simulink model "Simulation2"  (R2023b)
settings: Solver=VariableStepAuto  StartTime=0.0  StopTime=5  RelTol=1e-3
values from neighbouring files (symbols this model uses):
  Adj = Adj1'    [graph_plot.m]
  G = digraph(Adj)    [graph_plot.m]
undefined symbols (not defined in the file or in its folder): A, B, c, C, F, K, Ko, L1, x0_0, xi_0
libraries: simulink x7
settings Model: Creator=fedpa  LastModifiedBy=fedpa

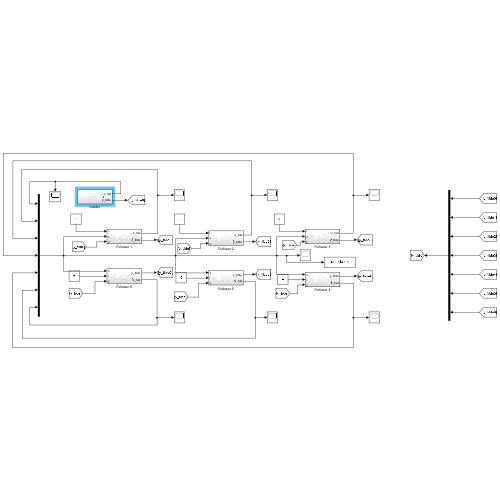
[thumbnail: Simulink's stored preview of the top-level diagram]
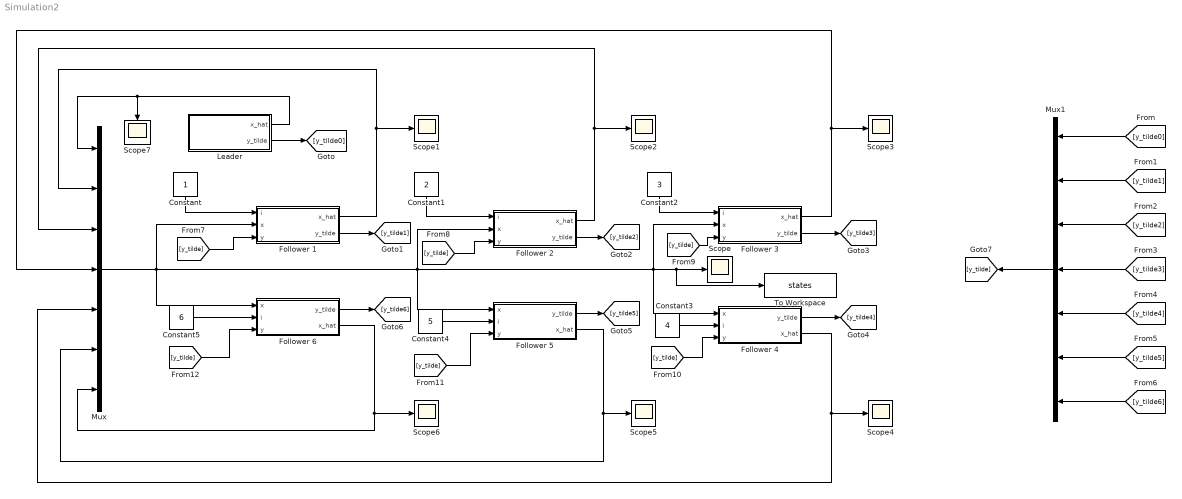
== system Simulation2 ==
  Constant : Constant
  Constant1 : Constant  Value=2
  Constant2 : Constant  Value=3
  Constant3 : Constant  Value=4
  Constant4 : Constant  Value=5
  Constant5 : Constant  Value=6
  Follower 1 : Subsystem
  Follower 2 : Subsystem
  Follower 3 : Subsystem
  Follower 4 : Subsystem
  Follower 5 : Subsystem
  Follower 6 : Subsystem
  Leader : Subsystem
  Mux : Mux  Inputs=7
  Mux1 : Mux  Inputs=7
  Scope{,1..7} (8 alike) : Scope
  To Workspace : ToWorkspace  VariableName=states  SaveFormat=Timeseries  SampleTime=-1
  wires:
  Follower 1/1(x_hat) -> Scope1/1, Mux/2
  Follower 2/1(x_hat) -> Scope2/1, Mux/3
  Follower 3/1(x_hat) -> Scope3/1, Mux/4
  Follower 6/2(x_hat) -> Scope6/1, Mux/7
  Follower 4/2(x_hat) -> Scope4/1, Mux/5
  Mux/1 -> To Workspace/1, Scope/1, Follower 4/1(x), Follower 3/2(x), Follower 5/1(x), Follower 2/2(x), Follower 6/1(x), Follower 1/2(x)
  Constant/1 -> Follower 1/1(i)
  Constant1/1 -> Follower 2/1(i)
  Constant2/1 -> Follower 3/1(i)
  Leader/1(x_hat) -> Scope7/1, Mux/1
  Leader/2(y_tilde) -> [y_tilde0]
  [y_tilde0] -> Mux1/1
  [y_tilde1] -> Mux1/2
  Follower 1/2(y_tilde) -> [y_tilde1]
  Follower 2/2(y_tilde) -> [y_tilde2]
  Follower 3/2(y_tilde) -> [y_tilde3]
  [y_tilde2] -> Mux1/3
  [y_tilde5] -> Mux1/6
  [y_tilde4] -> Mux1/5
  [y_tilde3] -> Mux1/4
  Follower 4/1(y_tilde) -> [y_tilde4]
  Follower 5/2(x_hat) -> Mux/6, Scope5/1
  Follower 5/1(y_tilde) -> [y_tilde5]
  Follower 6/1(y_tilde) -> [y_tilde6]
  [y_tilde6] -> Mux1/7
  Mux1/1 -> [y_tilde]
  [y_tilde] -> Follower 6/3(y)
  [y_tilde] -> Follower 5/3(y)
  [y_tilde] -> Follower 4/3(y)
  [y_tilde] -> Follower 3/3(y)
  [y_tilde] -> Follower 2/3(y)
  [y_tilde] -> Follower 1/3(y)
  Constant4/1 -> Follower 5/2(i)
  Constant5/1 -> Follower 6/2(i)
  Constant3/1 -> Follower 4/2(i)

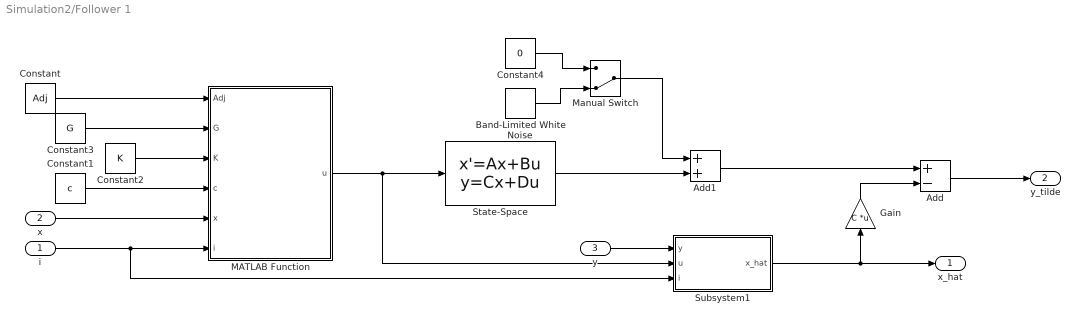
== system Simulation2/Follower 1 ==
  i : Inport
  x : Inport  Port=2
  y : Inport  Port=3
  Add : Sum  Inputs=+-
  Add1 : Sum
  Band-Limited White Noise : simulink/Sources/Band-Limited White Noise  Cov=dis  Ts=0.1  seed=[23341]
  Constant : Constant  Value=Adj  VectorParams1D=off
  Constant1 : Constant  Value=c
  Constant2 : Constant  Value=K  VectorParams1D=off
  Constant3 : Constant  Value=G
  Constant4 : Constant  Value=0
  Gain : Gain  Gain=C  Multiplication=Matrix(K*u)
  MATLAB Function : MATLAB Function  TreatAsAtomicUnit=on
  Manual Switch : ManualSwitch  CurrentSetting=0
  State-Space : StateSpace  A=A-B*Ko  B=B  C=C  D=0  InitialCondition=xi_0
  Subsystem1 : Subsystem
  x_hat : Outport
  y_tilde : Outport  Port=2
  wires:
  x/1 -> MATLAB Function/5(x)
  i/1 -> Subsystem1/3(i), MATLAB Function/6(i)
  Constant/1 -> MATLAB Function/1(Adj)
  Constant1/1 -> MATLAB Function/4(c)
  Constant2/1 -> MATLAB Function/3(K)
  Constant3/1 -> MATLAB Function/2(G)
  MATLAB Function/1(u) -> Subsystem1/2(u), State-Space/1
  Subsystem1/1(x_hat) -> x_hat/1, Gain/1
  Add/1 -> y_tilde/1
  y/1 -> Subsystem1/1(y)
  Gain/1 -> Add/2
  Add1/1 -> Add/1
  Constant4/1 -> Manual Switch/1
  Band-Limited White Noise/1 -> Manual Switch/2
  State-Space/1 -> Add1/2
  Manual Switch/1 -> Add1/1

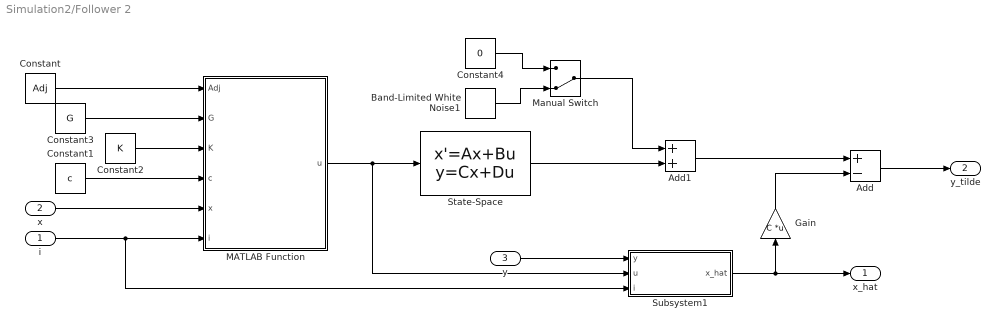
== system Simulation2/Follower 2 ==
  i : Inport
  x : Inport  Port=2
  y : Inport  Port=3
  Add : Sum  Inputs=+-
  Add1 : Sum
  Band-Limited White Noise1 : simulink/Sources/Band-Limited White Noise  Cov=dis  Ts=0.1  seed=[23341]
  Constant : Constant  Value=Adj  VectorParams1D=off
  Constant1 : Constant  Value=c
  Constant2 : Constant  Value=K  VectorParams1D=off
  Constant3 : Constant  Value=G
  Constant4 : Constant  Value=0
  Gain : Gain  Gain=C  Multiplication=Matrix(K*u)
  MATLAB Function : MATLAB Function  TreatAsAtomicUnit=on
  Manual Switch : ManualSwitch  CurrentSetting=0
  State-Space : StateSpace  A=A-B*Ko  B=B  C=C  D=0  InitialCondition=xi_0
  Subsystem1 : Subsystem
  x_hat : Outport
  y_tilde : Outport  Port=2
  wires:
  x/1 -> MATLAB Function/5(x)
  i/1 -> Subsystem1/3(i), MATLAB Function/6(i)
  Constant/1 -> MATLAB Function/1(Adj)
  Constant1/1 -> MATLAB Function/4(c)
  Constant2/1 -> MATLAB Function/3(K)
  Constant3/1 -> MATLAB Function/2(G)
  MATLAB Function/1(u) -> State-Space/1, Subsystem1/2(u)
  Subsystem1/1(x_hat) -> Gain/1, x_hat/1
  Add/1 -> y_tilde/1
  y/1 -> Subsystem1/1(y)
  Gain/1 -> Add/2
  Add1/1 -> Add/1
  Constant4/1 -> Manual Switch/1
  Band-Limited White Noise1/1 -> Manual Switch/2
  State-Space/1 -> Add1/2
  Manual Switch/1 -> Add1/1

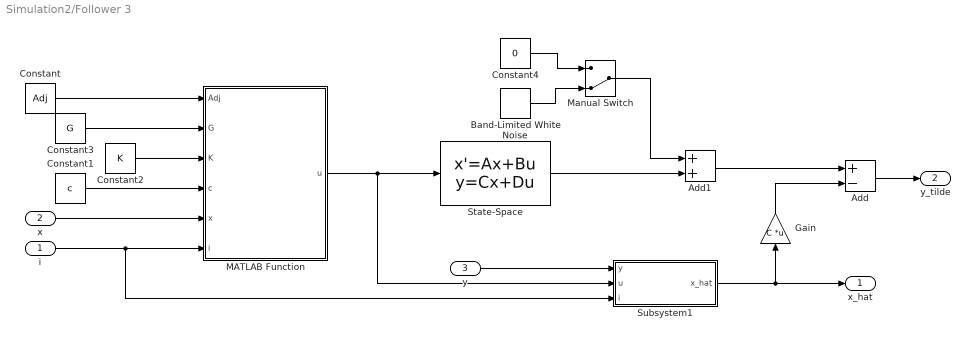
== system Simulation2/Follower 3 ==
  i : Inport
  x : Inport  Port=2
  y : Inport  Port=3
  Add : Sum  Inputs=+-
  Add1 : Sum
  Band-Limited White Noise : simulink/Sources/Band-Limited White Noise  Cov=dis  Ts=0.1  seed=[23341]
  Constant : Constant  Value=Adj  VectorParams1D=off
  Constant1 : Constant  Value=c
  Constant2 : Constant  Value=K  VectorParams1D=off
  Constant3 : Constant  Value=G
  Constant4 : Constant  Value=0
  Gain : Gain  Gain=C  Multiplication=Matrix(K*u)
  MATLAB Function : MATLAB Function  TreatAsAtomicUnit=on
  Manual Switch : ManualSwitch  CurrentSetting=0
  State-Space : StateSpace  A=A-B*Ko  B=B  C=C  D=0  InitialCondition=xi_0
  Subsystem1 : Subsystem
  x_hat : Outport
  y_tilde : Outport  Port=2
  wires:
  x/1 -> MATLAB Function/5(x)
  i/1 -> Subsystem1/3(i), MATLAB Function/6(i)
  Constant/1 -> MATLAB Function/1(Adj)
  Constant1/1 -> MATLAB Function/4(c)
  Constant2/1 -> MATLAB Function/3(K)
  Constant3/1 -> MATLAB Function/2(G)
  MATLAB Function/1(u) -> Subsystem1/2(u), State-Space/1
  Subsystem1/1(x_hat) -> Gain/1, x_hat/1
  Add/1 -> y_tilde/1
  y/1 -> Subsystem1/1(y)
  Gain/1 -> Add/2
  Add1/1 -> Add/1
  State-Space/1 -> Add1/2
  Constant4/1 -> Manual Switch/1
  Band-Limited White Noise/1 -> Manual Switch/2
  Manual Switch/1 -> Add1/1

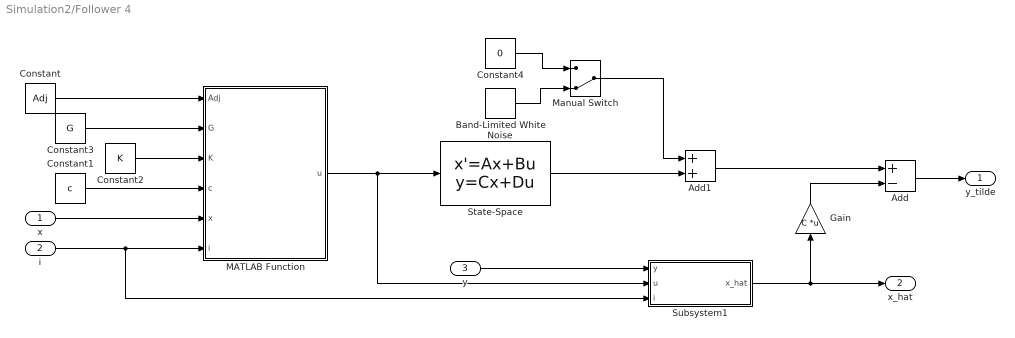
== system Simulation2/Follower 4 ==
  x : Inport
  i : Inport  Port=2
  y : Inport  Port=3
  Add : Sum  Inputs=+-
  Add1 : Sum
  Band-Limited White Noise : simulink/Sources/Band-Limited White Noise  Cov=dis  Ts=0.1  seed=[23341]
  Constant : Constant  Value=Adj  VectorParams1D=off
  Constant1 : Constant  Value=c
  Constant2 : Constant  Value=K  VectorParams1D=off
  Constant3 : Constant  Value=G
  Constant4 : Constant  Value=0
  Gain : Gain  Gain=C  Multiplication=Matrix(K*u)
  MATLAB Function : MATLAB Function  TreatAsAtomicUnit=on
  Manual Switch : ManualSwitch  CurrentSetting=0
  State-Space : StateSpace  A=A-B*Ko  B=B  C=C  D=0  InitialCondition=xi_0
  Subsystem1 : Subsystem
  y_tilde : Outport
  x_hat : Outport  Port=2
  wires:
  x/1 -> MATLAB Function/5(x)
  i/1 -> Subsystem1/3(i), MATLAB Function/6(i)
  Constant/1 -> MATLAB Function/1(Adj)
  Constant1/1 -> MATLAB Function/4(c)
  Constant2/1 -> MATLAB Function/3(K)
  Constant3/1 -> MATLAB Function/2(G)
  MATLAB Function/1(u) -> Subsystem1/2(u), State-Space/1
  Subsystem1/1(x_hat) -> Gain/1, x_hat/1
  Add/1 -> y_tilde/1
  y/1 -> Subsystem1/1(y)
  Gain/1 -> Add/2
  State-Space/1 -> Add1/2
  Add1/1 -> Add/1
  Constant4/1 -> Manual Switch/1
  Band-Limited White Noise/1 -> Manual Switch/2
  Manual Switch/1 -> Add1/1

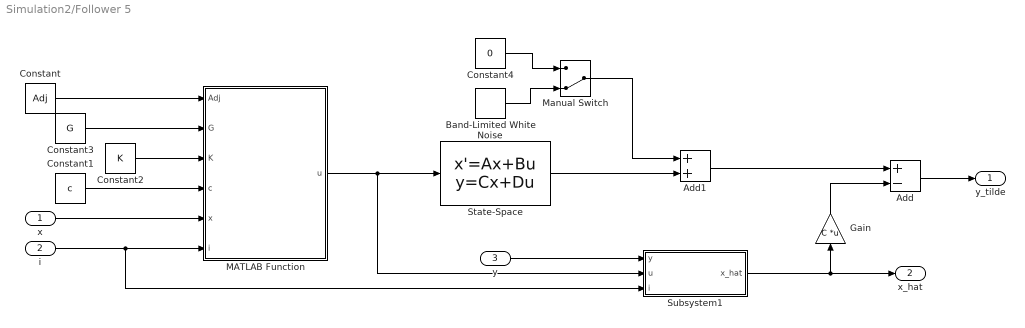
== system Simulation2/Follower 5 ==
  x : Inport
  i : Inport  Port=2
  y : Inport  Port=3
  Add : Sum  Inputs=+-
  Add1 : Sum
  Band-Limited White Noise : simulink/Sources/Band-Limited White Noise  Cov=dis  Ts=0.1  seed=[23341]
  Constant : Constant  Value=Adj  VectorParams1D=off
  Constant1 : Constant  Value=c
  Constant2 : Constant  Value=K  VectorParams1D=off
  Constant3 : Constant  Value=G
  Constant4 : Constant  Value=0
  Gain : Gain  Gain=C  Multiplication=Matrix(K*u)
  MATLAB Function : MATLAB Function  TreatAsAtomicUnit=on
  Manual Switch : ManualSwitch  CurrentSetting=0
  State-Space : StateSpace  A=A-B*Ko  B=B  C=C  D=0  InitialCondition=xi_0
  Subsystem1 : Subsystem
  y_tilde : Outport
  x_hat : Outport  Port=2
  wires:
  x/1 -> MATLAB Function/5(x)
  i/1 -> Subsystem1/3(i), MATLAB Function/6(i)
  Constant/1 -> MATLAB Function/1(Adj)
  Constant1/1 -> MATLAB Function/4(c)
  Constant2/1 -> MATLAB Function/3(K)
  Constant3/1 -> MATLAB Function/2(G)
  MATLAB Function/1(u) -> Subsystem1/2(u), State-Space/1
  Subsystem1/1(x_hat) -> Gain/1, x_hat/1
  Add/1 -> y_tilde/1
  y/1 -> Subsystem1/1(y)
  Gain/1 -> Add/2
  Add1/1 -> Add/1
  State-Space/1 -> Add1/2
  Constant4/1 -> Manual Switch/1
  Band-Limited White Noise/1 -> Manual Switch/2
  Manual Switch/1 -> Add1/1

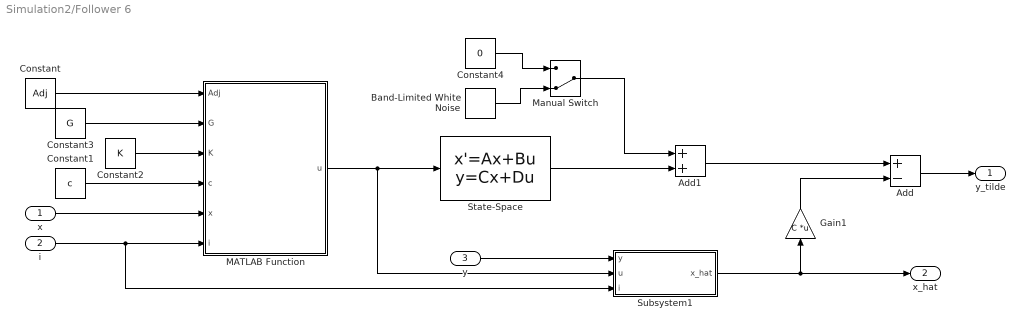
== system Simulation2/Follower 6 ==
  x : Inport
  i : Inport  Port=2
  y : Inport  Port=3
  Add : Sum  Inputs=+-
  Add1 : Sum
  Band-Limited White Noise : simulink/Sources/Band-Limited White Noise  Cov=dis  Ts=0.1  seed=[23341]
  Constant : Constant  Value=Adj  VectorParams1D=off
  Constant1 : Constant  Value=c
  Constant2 : Constant  Value=K  VectorParams1D=off
  Constant3 : Constant  Value=G
  Constant4 : Constant  Value=0
  Gain1 : Gain  Gain=C  Multiplication=Matrix(K*u)
  MATLAB Function : MATLAB Function  TreatAsAtomicUnit=on
  Manual Switch : ManualSwitch  CurrentSetting=0
  State-Space : StateSpace  A=A-B*Ko  B=B  C=C  D=0  InitialCondition=xi_0
  Subsystem1 : Subsystem
  y_tilde : Outport
  x_hat : Outport  Port=2
  wires:
  x/1 -> MATLAB Function/5(x)
  i/1 -> Subsystem1/3(i), MATLAB Function/6(i)
  Constant/1 -> MATLAB Function/1(Adj)
  Constant1/1 -> MATLAB Function/4(c)
  Constant2/1 -> MATLAB Function/3(K)
  Constant3/1 -> MATLAB Function/2(G)
  MATLAB Function/1(u) -> Subsystem1/2(u), State-Space/1
  Subsystem1/1(x_hat) -> Gain1/1, x_hat/1
  Add/1 -> y_tilde/1
  y/1 -> Subsystem1/1(y)
  Gain1/1 -> Add/2
  Add1/1 -> Add/1
  State-Space/1 -> Add1/2
  Constant4/1 -> Manual Switch/1
  Band-Limited White Noise/1 -> Manual Switch/2
  Manual Switch/1 -> Add1/1

== system Simulation2/Leader ==
  Add : Sum
  Add1 : Sum  Inputs=-+
  Band-Limited White Noise : simulink/Sources/Band-Limited White Noise  Cov=dis  Ts=0.1  seed=[23341]
  Constant : Constant  Value=0
  Gain : Gain  Gain=-Ko  Multiplication=Matrix(K*u)
  Gain1 : Gain  Gain=C  Multiplication=Matrix(K*u)
  Manual Switch : ManualSwitch
  Mux : Mux  Inputs=2
  State-Space : StateSpace  A=A  B=B  C=C  D=0  InitialCondition=x0_0
  State-Space1 : StateSpace  A=A-L1*C  B=[B L1]  C=eye(2)  D=zeros(2,2)  InitialCondition=0
  x_hat : Outport
  y_tilde : Outport  Port=2
  wires:
  Gain/1 -> State-Space/1, Mux/1
  State-Space1/1 -> x_hat/1, Gain1/1, Gain/1
  Add/1 -> Add1/2, Mux/2
  Manual Switch/1 -> Add/2
  Mux/1 -> State-Space1/1
  State-Space/1 -> Add/1
  Gain1/1 -> Add1/1
  Add1/1 -> y_tilde/1
  Constant/1 -> Manual Switch/1
  Band-Limited White Noise/1 -> Manual Switch/2

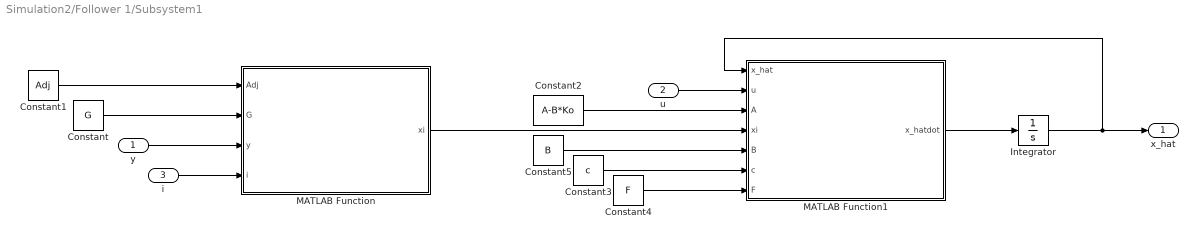
== system Simulation2/Follower 1/Subsystem1 ==
  y : Inport
  u : Inport  Port=2
  i : Inport  Port=3
  Constant : Constant  Value=G  VectorParams1D=off
  Constant1 : Constant  Value=Adj
  Constant2 : Constant  Value=A-B*Ko  VectorParams1D=off
  Constant3 : Constant  Value=c
  Constant4 : Constant  Value=F  VectorParams1D=off
  Constant5 : Constant  Value=B  VectorParams1D=off
  Integrator : Integrator  InitialCondition=[0 0]'
  MATLAB Function : MATLAB Function  TreatAsAtomicUnit=on
  MATLAB Function1 : MATLAB Function  TreatAsAtomicUnit=on
  x_hat : Outport
  wires:
  MATLAB Function1/1(x_hatdot) -> Integrator/1
  y/1 -> MATLAB Function/3(y)
  i/1 -> MATLAB Function/4(i)
  Constant/1 -> MATLAB Function/2(G)
  Constant1/1 -> MATLAB Function/1(Adj)
  MATLAB Function/1(xi) -> MATLAB Function1/4(xi)
  Constant2/1 -> MATLAB Function1/3(A)
  u/1 -> MATLAB Function1/2(u)
  Integrator/1 -> x_hat/1, MATLAB Function1/1(x_hat)
  Constant4/1 -> MATLAB Function1/7(F)
  Constant3/1 -> MATLAB Function1/6(c)
  Constant5/1 -> MATLAB Function1/5(B)

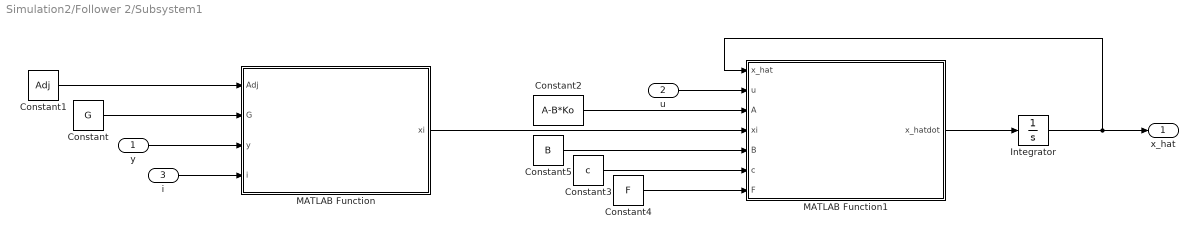
== system Simulation2/Follower 2/Subsystem1 ==
  y : Inport
  u : Inport  Port=2
  i : Inport  Port=3
  Constant : Constant  Value=G  VectorParams1D=off
  Constant1 : Constant  Value=Adj
  Constant2 : Constant  Value=A-B*Ko  VectorParams1D=off
  Constant3 : Constant  Value=c
  Constant4 : Constant  Value=F  VectorParams1D=off
  Constant5 : Constant  Value=B  VectorParams1D=off
  Integrator : Integrator  InitialCondition=[0 0]'
  MATLAB Function : MATLAB Function  TreatAsAtomicUnit=on
  MATLAB Function1 : MATLAB Function  TreatAsAtomicUnit=on
  x_hat : Outport
  wires:
  MATLAB Function1/1(x_hatdot) -> Integrator/1
  y/1 -> MATLAB Function/3(y)
  i/1 -> MATLAB Function/4(i)
  Constant/1 -> MATLAB Function/2(G)
  Constant1/1 -> MATLAB Function/1(Adj)
  MATLAB Function/1(xi) -> MATLAB Function1/4(xi)
  Constant2/1 -> MATLAB Function1/3(A)
  u/1 -> MATLAB Function1/2(u)
  Integrator/1 -> x_hat/1, MATLAB Function1/1(x_hat)
  Constant4/1 -> MATLAB Function1/7(F)
  Constant3/1 -> MATLAB Function1/6(c)
  Constant5/1 -> MATLAB Function1/5(B)

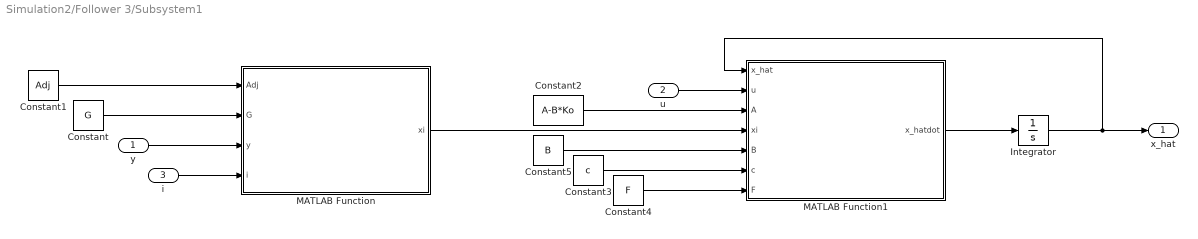
== system Simulation2/Follower 3/Subsystem1 ==
  y : Inport
  u : Inport  Port=2
  i : Inport  Port=3
  Constant : Constant  Value=G  VectorParams1D=off
  Constant1 : Constant  Value=Adj
  Constant2 : Constant  Value=A-B*Ko  VectorParams1D=off
  Constant3 : Constant  Value=c
  Constant4 : Constant  Value=F  VectorParams1D=off
  Constant5 : Constant  Value=B  VectorParams1D=off
  Integrator : Integrator  InitialCondition=[0 0]'
  MATLAB Function : MATLAB Function  TreatAsAtomicUnit=on
  MATLAB Function1 : MATLAB Function  TreatAsAtomicUnit=on
  x_hat : Outport
  wires:
  MATLAB Function1/1(x_hatdot) -> Integrator/1
  y/1 -> MATLAB Function/3(y)
  i/1 -> MATLAB Function/4(i)
  Constant/1 -> MATLAB Function/2(G)
  Constant1/1 -> MATLAB Function/1(Adj)
  MATLAB Function/1(xi) -> MATLAB Function1/4(xi)
  Constant2/1 -> MATLAB Function1/3(A)
  u/1 -> MATLAB Function1/2(u)
  Integrator/1 -> x_hat/1, MATLAB Function1/1(x_hat)
  Constant4/1 -> MATLAB Function1/7(F)
  Constant3/1 -> MATLAB Function1/6(c)
  Constant5/1 -> MATLAB Function1/5(B)

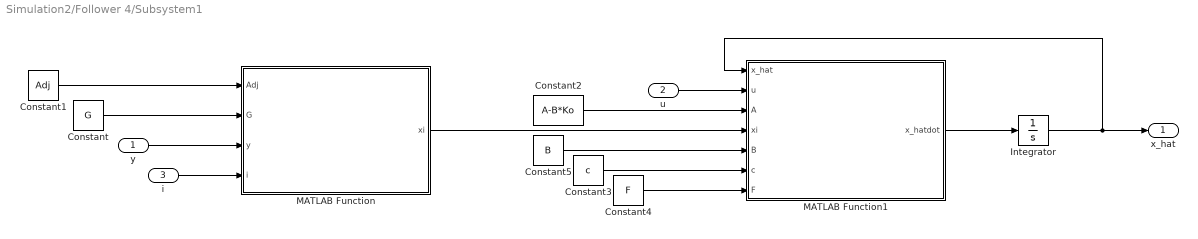
== system Simulation2/Follower 4/Subsystem1 ==
  y : Inport
  u : Inport  Port=2
  i : Inport  Port=3
  Constant : Constant  Value=G  VectorParams1D=off
  Constant1 : Constant  Value=Adj
  Constant2 : Constant  Value=A-B*Ko  VectorParams1D=off
  Constant3 : Constant  Value=c
  Constant4 : Constant  Value=F  VectorParams1D=off
  Constant5 : Constant  Value=B  VectorParams1D=off
  Integrator : Integrator  InitialCondition=[0 0]'
  MATLAB Function : MATLAB Function  TreatAsAtomicUnit=on
  MATLAB Function1 : MATLAB Function  TreatAsAtomicUnit=on
  x_hat : Outport
  wires:
  MATLAB Function1/1(x_hatdot) -> Integrator/1
  y/1 -> MATLAB Function/3(y)
  i/1 -> MATLAB Function/4(i)
  Constant/1 -> MATLAB Function/2(G)
  Constant1/1 -> MATLAB Function/1(Adj)
  MATLAB Function/1(xi) -> MATLAB Function1/4(xi)
  Constant2/1 -> MATLAB Function1/3(A)
  u/1 -> MATLAB Function1/2(u)
  Integrator/1 -> x_hat/1, MATLAB Function1/1(x_hat)
  Constant4/1 -> MATLAB Function1/7(F)
  Constant3/1 -> MATLAB Function1/6(c)
  Constant5/1 -> MATLAB Function1/5(B)

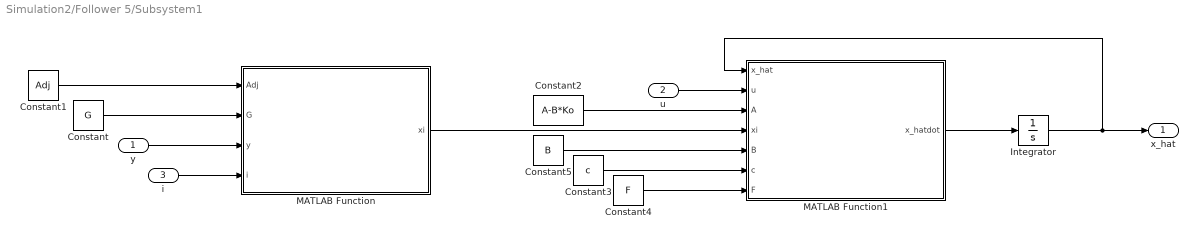
== system Simulation2/Follower 5/Subsystem1 ==
  y : Inport
  u : Inport  Port=2
  i : Inport  Port=3
  Constant : Constant  Value=G  VectorParams1D=off
  Constant1 : Constant  Value=Adj
  Constant2 : Constant  Value=A-B*Ko  VectorParams1D=off
  Constant3 : Constant  Value=c
  Constant4 : Constant  Value=F  VectorParams1D=off
  Constant5 : Constant  Value=B  VectorParams1D=off
  Integrator : Integrator  InitialCondition=[0 0]'
  MATLAB Function : MATLAB Function  TreatAsAtomicUnit=on
  MATLAB Function1 : MATLAB Function  TreatAsAtomicUnit=on
  x_hat : Outport
  wires:
  MATLAB Function1/1(x_hatdot) -> Integrator/1
  y/1 -> MATLAB Function/3(y)
  i/1 -> MATLAB Function/4(i)
  Constant/1 -> MATLAB Function/2(G)
  Constant1/1 -> MATLAB Function/1(Adj)
  MATLAB Function/1(xi) -> MATLAB Function1/4(xi)
  Constant2/1 -> MATLAB Function1/3(A)
  u/1 -> MATLAB Function1/2(u)
  Integrator/1 -> x_hat/1, MATLAB Function1/1(x_hat)
  Constant4/1 -> MATLAB Function1/7(F)
  Constant3/1 -> MATLAB Function1/6(c)
  Constant5/1 -> MATLAB Function1/5(B)

== system Simulation2/Follower 6/Subsystem1 ==
  y : Inport
  u : Inport  Port=2
  i : Inport  Port=3
  Constant : Constant  Value=G  VectorParams1D=off
  Constant1 : Constant  Value=Adj
  Constant2 : Constant  Value=A-B*Ko  VectorParams1D=off
  Constant3 : Constant  Value=c
  Constant4 : Constant  Value=F  VectorParams1D=off
  Constant5 : Constant  Value=B  VectorParams1D=off
  Integrator : Integrator  InitialCondition=[0 0]'
  MATLAB Function : MATLAB Function  TreatAsAtomicUnit=on
  MATLAB Function1 : MATLAB Function  TreatAsAtomicUnit=on
  x_hat : Outport
  wires:
  MATLAB Function1/1(x_hatdot) -> Integrator/1
  y/1 -> MATLAB Function/3(y)
  i/1 -> MATLAB Function/4(i)
  Constant/1 -> MATLAB Function/2(G)
  Constant1/1 -> MATLAB Function/1(Adj)
  MATLAB Function/1(xi) -> MATLAB Function1/4(xi)
  Constant2/1 -> MATLAB Function1/3(A)
  u/1 -> MATLAB Function1/2(u)
  Integrator/1 -> x_hat/1, MATLAB Function1/1(x_hat)
  Constant4/1 -> MATLAB Function1/7(F)
  Constant3/1 -> MATLAB Function1/6(c)
  Constant5/1 -> MATLAB Function1/5(B)

== matlab function Simulation2/Follower 5/MATLAB Function ==
  data: Adj input; u output; G input; K input; c input; x input; i input
function u = fcn(Adj, G, K, c, x, i)
    epsi = zeros(2,1);
    for j=1:6 
        epsi = epsi + Adj(i,j)*(x(j*2+1:j*2+2)-x(i*2+1:i*2+2));
    end
    epsi = epsi + G(i,i)*(x(1:2)-x(i*2+1:i*2+2));

    u = c*K*epsi;
end

== matlab function Simulation2/Follower 5/Subsystem1/MATLAB Function ==
  data: Adj input; xi output; G input; y input; i input
function xi = fcn(Adj, G, y, i)
    xi = 0;
    for j=1:6 
        xi = xi + Adj(i,j)*(y(j+1)-y(i+1));
    end
    xi = xi + G(i,i)*(y(1)-y(i+1));
end

== matlab function Simulation2/Follower 5/Subsystem1/MATLAB Function1 ==
  data: x_hat input; u input; A input; x_hatdot output; xi input; B input; c input; F input
function x_hatdot = neighborObserver(x_hat,u,A,xi,B,c,F)
    x_hatdot = A*x_hat+B*u-c*F*xi;
end

== matlab function Simulation2/Follower 1/MATLAB Function ==
  data: Adj input; u output; G input; K input; c input; x input; i input
function u = fcn(Adj, G, K, c, x, i)
    epsi = zeros(2,1);
    for j=1:6 
        epsi = epsi + Adj(i,j)*(x(j*2+1:j*2+2)-x(i*2+1:i*2+2));
    end
    epsi = epsi + G(i,i)*(x(1:2)-x(i*2+1:i*2+2));

    u = c*K*epsi;
end

== matlab function Simulation2/Follower 6/MATLAB Function ==
  data: Adj input; u output; G input; K input; c input; x input; i input
function u = fcn(Adj, G, K, c, x, i)
    epsi = zeros(2,1);
    for j=1:6 
        epsi = epsi + Adj(i,j)*(x(j*2+1:j*2+2)-x(i*2+1:i*2+2));
    end
    epsi = epsi + G(i,i)*(x(1:2)-x(i*2+1:i*2+2));

    u = c*K*epsi;
end

== matlab function Simulation2/Follower 1/Subsystem1/MATLAB Function1 ==
  data: x_hat input; u input; A input; x_hatdot output; xi input; B input; c input; F input
function x_hatdot = neighborObserver(x_hat,u,A,xi,B,c,F)
    x_hatdot = A*x_hat+B*u-c*F*xi;
end

== matlab function Simulation2/Follower 6/Subsystem1/MATLAB Function ==
  data: Adj input; xi output; G input; y input; i input
function xi = fcn(Adj, G, y, i)
    xi = 0;
    for j=1:6 
        xi = xi + Adj(i,j)*(y(j+1)-y(i+1));
    end
    xi = xi + G(i,i)*(y(1)-y(i+1));
end

== matlab function Simulation2/Follower 6/Subsystem1/MATLAB Function1 ==
  data: x_hat input; u input; A input; x_hatdot output; xi input; B input; c input; F input
function x_hatdot = neighborObserver(x_hat,u,A,xi,B,c,F)
    x_hatdot = A*x_hat+B*u-c*F*xi;
end

== matlab function Simulation2/Follower 2/MATLAB Function ==
  data: Adj input; u output; G input; K input; c input; x input; i input
function u = fcn(Adj, G, K, c, x, i)
    epsi = zeros(2,1);
    for j=1:6 
        epsi = epsi + Adj(i,j)*(x(j*2+1:j*2+2)-x(i*2+1:i*2+2));
    end
    epsi = epsi + G(i,i)*(x(1:2)-x(i*2+1:i*2+2));

    u = c*K*epsi;
end

== matlab function Simulation2/Follower 2/Subsystem1/MATLAB Function ==
  data: Adj input; xi output; G input; y input; i input
function xi = fcn(Adj, G, y, i)
    xi = 0;
    for j=1:6 
        xi = xi + Adj(i,j)*(y(j+1)-y(i+1));
    end
    xi = xi + G(i,i)*(y(1)-y(i+1));
end

== matlab function Simulation2/Follower 2/Subsystem1/MATLAB Function1 ==
  data: x_hat input; u input; A input; x_hatdot output; xi input; B input; c input; F input
function x_hatdot = neighborObserver(x_hat,u,A,xi,B,c,F)
    x_hatdot = A*x_hat+B*u-c*F*xi;
end

== matlab function Simulation2/Follower 1/Subsystem1/MATLAB Function ==
  data: Adj input; xi output; G input; y input; i input
function xi = fcn(Adj, G, y, i)
    xi = 0;
    for j=1:6 
        xi = xi + Adj(i,j)*(y(j+1)-y(i+1));
    end
    xi = xi + G(i,i)*(y(1)-y(i+1));
end

== matlab function Simulation2/Follower 3/MATLAB Function ==
  data: Adj input; u output; G input; K input; c input; x input; i input
function u = fcn(Adj, G, K, c, x, i)
    epsi = zeros(2,1);
    for j=1:6 
        epsi = epsi + Adj(i,j)*(x(j*2+1:j*2+2)-x(i*2+1:i*2+2));
    end
    epsi = epsi + G(i,i)*(x(1:2)-x(i*2+1:i*2+2));

    u = c*K*epsi;
end

== matlab function Simulation2/Follower 3/Subsystem1/MATLAB Function ==
  data: Adj input; xi output; G input; y input; i input
function xi = fcn(Adj, G, y, i)
    xi = 0;
    for j=1:6 
        xi = xi + Adj(i,j)*(y(j+1)-y(i+1));
    end
    xi = xi + G(i,i)*(y(1)-y(i+1));
end

== matlab function Simulation2/Follower 3/Subsystem1/MATLAB Function1 ==
  data: x_hat input; u input; A input; x_hatdot output; xi input; B input; c input; F input
function x_hatdot = neighborObserver(x_hat,u,A,xi,B,c,F)
    x_hatdot = A*x_hat+B*u-c*F*xi;
end

== matlab function Simulation2/Follower 4/MATLAB Function ==
  data: Adj input; u output; G input; K input; c input; x input; i input
function u = fcn(Adj, G, K, c, x, i)
    epsi = zeros(2,1);
    for j=1:6 
        epsi = epsi + Adj(i,j)*(x(j*2+1:j*2+2)-x(i*2+1:i*2+2));
    end
    epsi = epsi + G(i,i)*(x(1:2)-x(i*2+1:i*2+2));

    u = c*K*epsi;
end

== matlab function Simulation2/Follower 4/Subsystem1/MATLAB Function ==
  data: Adj input; xi output; G input; y input; i input
function xi = fcn(Adj, G, y, i)
    xi = 0;
    for j=1:6 
        xi = xi + Adj(i,j)*(y(j+1)-y(i+1));
    end
    xi = xi + G(i,i)*(y(1)-y(i+1));
end

== matlab function Simulation2/Follower 4/Subsystem1/MATLAB Function1 ==
  data: x_hat input; u input; A input; x_hatdot output; xi input; B input; c input; F input
function x_hatdot = neighborObserver(x_hat,u,A,xi,B,c,F)
    x_hatdot = A*x_hat+B*u-c*F*xi;
end
